simulink model "T7_R2021a"  (R2022a)
settings: Solver=FixedStepAuto  StartTime=0.0  StopTime=10  FixedStep=Ts  RelTol=1e-10  AbsTol=1e-10
model workspace (MATLAB code in the model file):
  | %% Electrical parameters of PMSM motor
  | 
  | P_N = 530; % [W]
  | I_N = 1.5; % [A] (rms)
  | U_N = 220; % [V] (rms, line to line)
  | n_N = 4000; % [rpm]
  | PF_N = 0.9925;
  | n_p=2;
  | V_max = 400; %[V] (rms, line to line)
  | t_r_ref = 1e-3;
  | J = 0.384e-4*5; %kg.m^2
  | 
  | 
  | % Calculations:
  | 
  | % Question 1:
  | w_N = n_N*2*pi/60;
  | psi_R = 20*P_N/(sqrt(2)*pi*n_p*I_N*n_N);
  | L_s = 10*sqrt(3)*U_N*sin(acos(PF_N))/(n_p*n_N*pi*I_N);
  | R_s = sqrt(3)*U_N*PF_N/(3*I_N)-P_N/(3*I_N^2);
  | %% Current Controller
  | Ts = 1e-4;
  | T_L = 0;
  | t_r = 1e-3;
  | w_BW = log(9)/t_r;
  | %E_hat = 1i*w*Psi_R;
  | L_s_hat = 0.010;
  | R_s_hat = 4;
  | R_a = w_BW*L_s_hat - R_s_hat;
  | ki = w_BW*(R_s_hat+R_a);
  | kp = w_BW*L_s_hat;
undefined symbols (not defined in the file or in its folder): b, b_hat, I_max, J_hat, L_M, L_M_hat, L_sigma, L_sigma_hat, magnitude, omega_1_N, psi_R_hat, psi_ref, R_hat, R_R, R_R_hat, V_base, V_LL, w_BWs
libraries: simulink x2
settings Model: Creator=martin  LastModifiedBy=Katrine
settings ModelReferenceCC: EnableRefExpFcnMdlSchedulingChecks=off
settings RTWCC: Description=Generic Real-Time Target

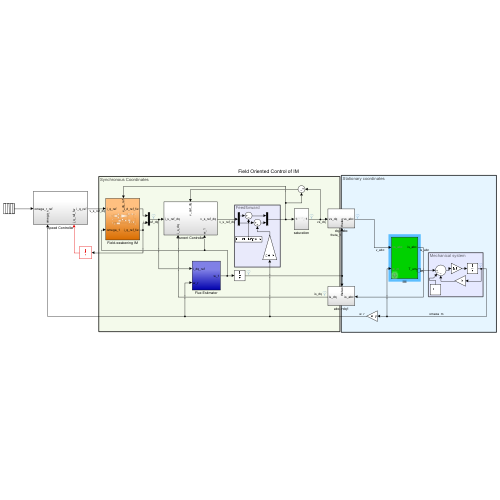
[thumbnail: Simulink's stored preview of the top-level diagram]
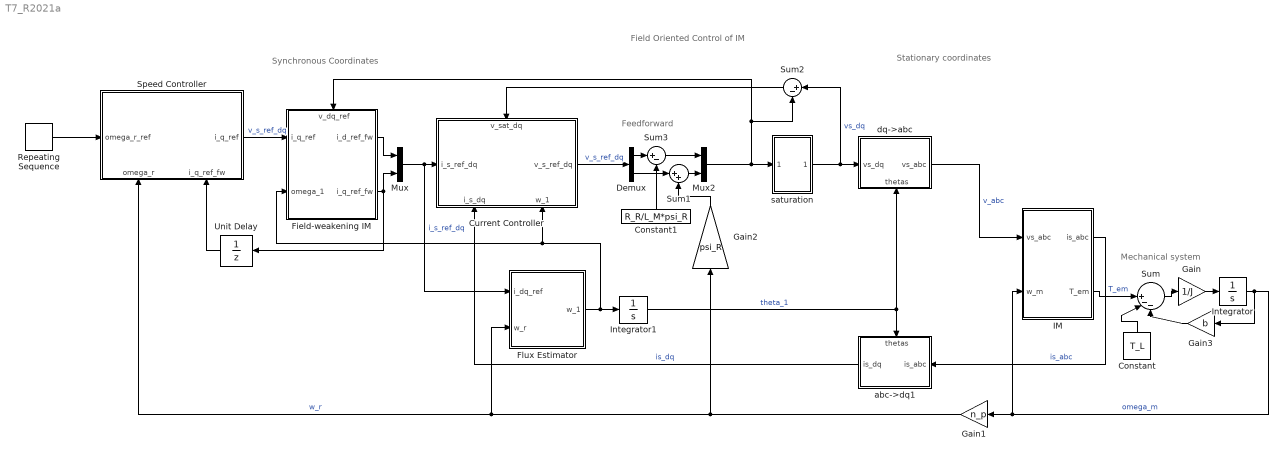
== system T7_R2021a ==
  note: Synchronous Coordinates
  note: Stationary coordinates
  note: Field Oriented Control of IM
  note: Mechanical system
  note: Feedforward
  Constant : Constant  Value=T_L
  Constant1 : Constant  Value=R_R/L_M*psi_R
  Current Controller : Subsystem
      settings: PortSchema="{\"entries\":[{\"content\":{\"sides\":[{\"content\":{\"connectorIds\":[\"In1\"]},\"type\":\"ConnectorPlacement.EquallySpacedRectSide\",\"uuid\":\"97c548b6-6990-4323-a853-1e64e742285c\"},{\"content\":{\"connectorIds\":[\"Out1\"],\"side\":\"RIGHT\"},\"type\":\"ConnectorPlacement.EquallySpacedRectSide\",\"uuid\":\"cacb7644-0a67-4de4-9bb2-887734fe331a\"},{\"content\":{\"connectorIds\":[\"In2\"],\"side\":\"TOP\"},\"type\":\"ConnectorPlacement.EquallySpacedRectSide\",\"uuid\":\"a20c1423-7334-426c-a525-8bdb26886bc3\"},{\"content\":{\"connectorIds\":[\"In3\",\"In4\"],\"side\":\"BOTTOM\"},\"type\":\"ConnectorPlacement.EquallySpacedRectSide\",\"uuid\":\"b9821709-22a3-4c1b-ad46-11760bdb190f\"}]},\"type\":\"ConnectorPlacement.EquallySpacedConnector\",\"uuid\":\"74caaff1-86aa-4f34-8e3a-31d84a5552f1\"}],\"packageUris\":[\"http://schema.mathworks.com/mf0/Connector/R2020b\"],\"version\":\"1.0\"}"
  Demux : Demux  Outputs=2
  Field-weakening IM : Subsystem
      settings: PortSchema="{\"entries\":[{\"content\":{\"sides\":[{\"content\":{\"connectorIds\":[\"In1\",\"In2\"]},\"type\":\"ConnectorPlacement.EquallySpacedRectSide\",\"uuid\":\"aee381d7-3a71-45d0-966d-7af6601206c5\"},{\"content\":{\"connectorIds\":[\"Out1\",\"Out2\"],\"side\":\"RIGHT\"},\"type\":\"ConnectorPlacement.EquallySpacedRectSide\",\"uuid\":\"b4f04b7a-b16d-4ae2-8d18-1ccf45d54418\"},{\"content\":{\"connectorIds\":[\"In3\"],\"side\":\"TOP\"},\"type\":\"ConnectorPlacement.EquallySpacedRectSide\",\"uuid\":\"7d29b16c-0908-4291-9b7c-a89871d4912d\"}]},\"type\":\"ConnectorPlacement.EquallySpacedConnector\",\"uuid\":\"28c927f9-c9f1-4063-8a99-a2da52e20e9b\"}],\"packageUris\":[\"http://schema.mathworks.com/mf0/Connector/R2020b\"],\"version\":\"1.0\"}"
  Flux Estimator : Subsystem
  Gain : Gain  Gain=1/J
  Gain1 : Gain  Gain=n_p
  Gain2 : Gain  Gain=psi_R
  Gain3 : Gain  Gain=b
  IM : Subsystem  mask{R_s=0.5, L_sig=6e-3, R_R=0.312, n_p=1, L_M=0.1}
      mask prompts: R_s "Stator resistance Rs (ohm)"; L_sig "Total leakage inductance L_sig (H)"; R_R "Rotor resistance R_R ( Ohm)"; n_p "Number of pole pairs n_p"; L_M "Magnetising inductance L_M (H)"
      mask help: dynamic model of IM
  Integrator : Integrator  InitialCondition=1337/n_p
  Integrator1 : Integrator
  Mux : Mux  Inputs=2
  Mux2 : Mux  Inputs=2
  Repeating Sequence : simulink/Sources/Repeating Sequence  rep_seq_t=[0 Ts*1e3 5 5+Ts*1e3 10]*1e-3  rep_seq_y=[4.3 4.3 4.3 1 1]
  Speed Controller : Subsystem
      settings: PortSchema="{\"entries\":[{\"content\":{\"sides\":[{\"content\":{\"connectorIds\":[\"In1\"]},\"type\":\"ConnectorPlacement.EquallySpacedRectSide\",\"uuid\":\"97c548b6-6990-4323-a853-1e64e742285c\"},{\"content\":{\"connectorIds\":[\"Out1\"],\"side\":\"RIGHT\"},\"type\":\"ConnectorPlacement.EquallySpacedRectSide\",\"uuid\":\"cacb7644-0a67-4de4-9bb2-887734fe331a\"},{\"content\":{\"connectorIds\":[],\"side\":\"TOP\"},\"type\":\"ConnectorPlacement.EquallySpacedRectSide\",\"uuid\":\"a20c1423-7334-426c-a525-8bdb26886bc3\"},{\"content\":{\"connectorIds\":[\"In2\",\"In3\"],\"side\":\"BOTTOM\"},\"type\":\"ConnectorPlacement.EquallySpacedRectSide\",\"uuid\":\"b9821709-22a3-4c1b-ad46-11760bdb190f\"}]},\"type\":\"ConnectorPlacement.EquallySpacedConnector\",\"uuid\":\"74caaff1-86aa-4f34-8e3a-31d84a5552f1\"}],\"packageUris\":[\"http://schema.mathworks.com/mf0/Connector/R2020b\"],\"version\":\"1.0\"}"
  Sum : Sum  Inputs=||+--
  Sum1 : Sum  Inputs=|++
  Sum2 : Sum  Inputs=|+-
  Sum3 : Sum  Inputs=|+-
  Unit Delay : UnitDelay  InitialCondition=I_max  SampleTime=-1  HasFrameUpgradeWarning=on
  abc->dq1 : Subsystem
      settings: PortSchema="{\"entries\":[{\"content\":{\"sides\":[{\"content\":{\"connectorIds\":[\"In1\"]},\"type\":\"ConnectorPlacement.EquallySpacedRectSide\",\"uuid\":\"c3863cce-4a98-427c-9e63-89298f679a84\"},{\"content\":{\"connectorIds\":[\"Out1\"],\"side\":\"RIGHT\"},\"type\":\"ConnectorPlacement.EquallySpacedRectSide\",\"uuid\":\"ae3c4991-ab62-4114-9bee-e9a7348a29ce\"},{\"content\":{\"connectorIds\":[\"In2\"],\"side\":\"TOP\"},\"type\":\"ConnectorPlacement.EquallySpacedRectSide\",\"uuid\":\"fea582b6-68e0-450b-8231-0f2cf258215e\"},{\"content\":{\"connectorIds\":[],\"side\":\"BOTTOM\"},\"type\":\"ConnectorPlacement.EquallySpacedRectSide\",\"uuid\":\"4cb5cb50-d1c5-41cc-b580-d3f7a61a133b\"}]},\"type\":\"ConnectorPlacement.EquallySpacedConnector\",\"uuid\":\"936995e1-3667-4d5a-83ac-5ed23eb7cec5\"}],\"packageUris\":[\"http://schema.mathworks.com/mf0/Connector/R2020b\"],\"version\":\"1.0\"}"
  dq->abc : Subsystem
      settings: PortSchema="{\"entries\":[{\"content\":{\"sides\":[{\"content\":{\"connectorIds\":[\"In1\"]},\"type\":\"ConnectorPlacement.EquallySpacedRectSide\",\"uuid\":\"c3863cce-4a98-427c-9e63-89298f679a84\"},{\"content\":{\"connectorIds\":[\"Out1\"],\"side\":\"RIGHT\"},\"type\":\"ConnectorPlacement.EquallySpacedRectSide\",\"uuid\":\"ae3c4991-ab62-4114-9bee-e9a7348a29ce\"},{\"content\":{\"connectorIds\":[],\"side\":\"TOP\"},\"type\":\"ConnectorPlacement.EquallySpacedRectSide\",\"uuid\":\"fea582b6-68e0-450b-8231-0f2cf258215e\"},{\"content\":{\"connectorIds\":[\"In2\"],\"side\":\"BOTTOM\"},\"type\":\"ConnectorPlacement.EquallySpacedRectSide\",\"uuid\":\"09df17c4-38be-4fcd-b44b-abaf9d5b2651\"}]},\"type\":\"ConnectorPlacement.EquallySpacedConnector\",\"uuid\":\"936995e1-3667-4d5a-83ac-5ed23eb7cec5\"}],\"packageUris\":[\"http://schema.mathworks.com/mf0/Connector/R2020b\"],\"version\":\"1.0\"}"
  saturation : Subsystem
  wires:
  dq->abc/1(vs_abc) -> IM/1(vs_abc)  "v_abc"
  Sum/1 -> Gain/1
  Gain/1 -> Integrator/1
  Integrator/1 -> Gain3/1, IM/2(w_m), Gain1/1  "omega_m"
  IM/2(T_em) -> Sum/1  "T_em"
  Constant/1 -> Sum/2
  IM/1(is_abc) -> abc->dq1/1(is_abc)  "is_abc"
  Integrator1/1 -> dq->abc/2(thetas), abc->dq1/2(thetas)  "theta_1"
  abc->dq1/1(is_dq) -> Current Controller/3(i_s_dq)  "is_dq"
  Mux/1 -> Flux Estimator/1(i_dq_ref), Current Controller/1(i_s_ref_dq)  "i_s_ref_dq"
  Current Controller/1(v_s_ref_dq) -> Demux/1  "v_s_ref_dq"
  Demux/2 -> Sum1/1
  Sum1/1 -> Mux2/2
  saturation/1(Out1) -> Sum2/1, dq->abc/1(vs_dq)  "vs_dq"
  Gain2/1 -> Sum1/2
  Sum2/1 -> Current Controller/2(v_sat_dq)
  Flux Estimator/1(w_1) -> Field-weakening IM/2(omega_1), Current Controller/4(w_1), Integrator1/1
  Gain1/1 -> Speed Controller/2(omega_r), Flux Estimator/2(w_r), Gain2/1  "w_r"
  Demux/1 -> Sum3/1
  Sum3/1 -> Mux2/1
  Constant1/1 -> Sum3/2
  Field-weakening IM/1(i_d_ref_fw) -> Mux/1
  Field-weakening IM/2(i_q_ref_fw) -> Unit Delay/1, Mux/2
  Mux2/1 -> Field-weakening IM/3(v_dq_ref), Sum2/2, saturation/1(In1)
  Gain3/1 -> Sum/3
  Speed Controller/1(i_q_ref) -> Field-weakening IM/1(i_q_ref)  "v_s_ref_dq"
  Repeating Sequence/1 -> Speed Controller/1(omega_r_ref)
  Unit Delay/1 -> Speed Controller/3(i_q_ref_fw)

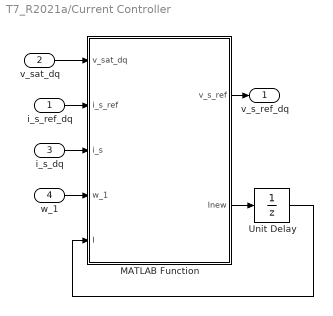
== system T7_R2021a/Current Controller ==
  i_s_ref_dq : Inport
  v_sat_dq : Inport  Port=2
  i_s_dq : Inport  Port=3
  w_1 : Inport  Port=4
  MATLAB Function : MATLAB Function  TreatAsAtomicUnit=on
  Unit Delay : UnitDelay  SampleTime=-1  HasFrameUpgradeWarning=on
  v_s_ref_dq : Outport  PortDimensions=2
  wires:
  MATLAB Function/2(Inew) -> Unit Delay/1
  i_s_ref_dq/1 -> MATLAB Function/2(i_s_ref)
  w_1/1 -> MATLAB Function/4(w_1)
  i_s_dq/1 -> MATLAB Function/3(i_s)
  Unit Delay/1 -> MATLAB Function/5(I)
  MATLAB Function/1(v_s_ref) -> v_s_ref_dq/1
  v_sat_dq/1 -> MATLAB Function/1(v_sat_dq)

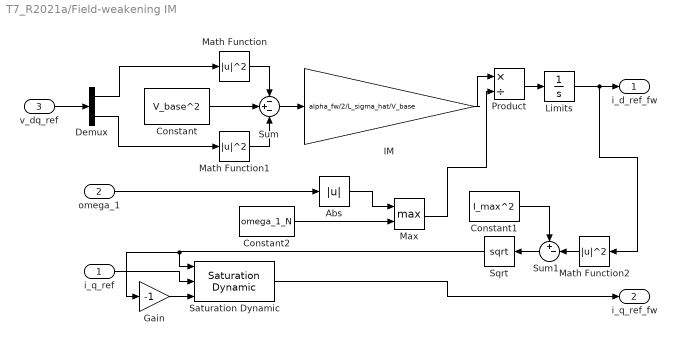
== system T7_R2021a/Field-weakening IM ==
  i_q_ref : Inport
  omega_1 : Inport  Port=2
  v_dq_ref : Inport  Port=3
  Abs : Abs  SaturateOnIntegerOverflow=off
  Constant : Constant  Value=V_base^2
  Constant1 : Constant  Value=I_max^2
  Constant2 : Constant  Value=omega_1_N
  Demux : Demux  Outputs=2
  Gain : Gain  Gain=-1
  IM : Gain  Gain=alpha_fw/2/L_sigma_hat/V_base
  Limits : Integrator  LimitOutput=on  UpperSaturationLimit=psi_ref/L_M_hat  LowerSaturationLimit=0.1*psi_ref/L_M_hat
  Math Function : Math  Operator=magnitude^2
  Math Function1 : Math  Operator=magnitude^2
  Math Function2 : Math  Operator=magnitude^2
  Max : MinMax  Function=max  Inputs=2
  Product : Product  Inputs=*/
  Saturation Dynamic : simulink/Discontinuities/Saturation Dynamic  OutMin=[]  OutMax=[]  OutDataTypeStr=Inherit: Same as second input  OutDataType=fixdt(1, 16)  OutScaling=2^-10  DoSatur=off
  Sqrt : Sqrt
  Sum : Sum  Inputs=-+-
  Sum1 : Sum  Inputs=+-|
  i_d_ref_fw : Outport
  i_q_ref_fw : Outport  Port=2
  wires:
  i_q_ref/1 -> Saturation Dynamic/2
  Constant/1 -> Sum/2
  Math Function/1 -> Sum/1
  Math Function1/1 -> Sum/3
  Sum/1 -> IM/1
  IM/1 -> Product/1
  omega_1/1 -> Abs/1
  Abs/1 -> Max/1
  Max/1 -> Product/2
  Product/1 -> Limits/1
  Limits/1 -> i_d_ref_fw/1, Math Function2/1
  Math Function2/1 -> Sum1/2
  Constant1/1 -> Sum1/1
  Sum1/1 -> Sqrt/1
  Sqrt/1 -> Gain/1, Saturation Dynamic/1
  Gain/1 -> Saturation Dynamic/3
  Saturation Dynamic/1 -> i_q_ref_fw/1
  Constant2/1 -> Max/2
  v_dq_ref/1 -> Demux/1
  Demux/1 -> Math Function/1
  Demux/2 -> Math Function1/1

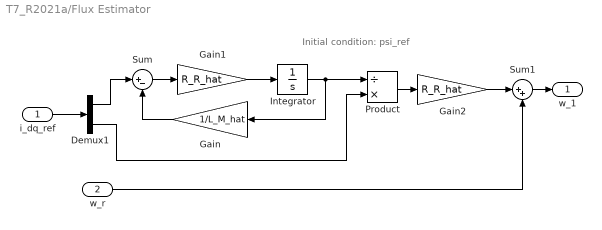
== system T7_R2021a/Flux Estimator ==
  note: Initial condition: psi_ref
  i_dq_ref : Inport
  w_r : Inport  Port=2
  Demux1 : Demux  Outputs=2
  Gain : Gain  Gain=1/L_M_hat
  Gain1 : Gain  Gain=R_R_hat
  Gain2 : Gain  Gain=R_R_hat
  Integrator : Integrator  InitialCondition=psi_ref
  Product : Product  Inputs=/*
  Sum : Sum  Inputs=|+-
  Sum1 : Sum  Inputs=|++
  w_1 : Outport
  wires:
  w_r/1 -> Sum1/2
  Sum1/1 -> w_1/1
  Gain2/1 -> Sum1/1
  Product/1 -> Gain2/1
  Demux1/2 -> Product/2
  Gain1/1 -> Integrator/1
  Sum/1 -> Gain1/1
  Gain/1 -> Sum/2
  Integrator/1 -> Gain/1, Product/1
  i_dq_ref/1 -> Demux1/1
  Demux1/1 -> Sum/1

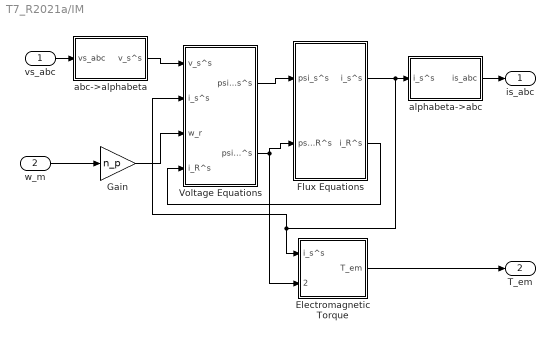
== system T7_R2021a/IM ==
  vs_abc : Inport
  w_m : Inport  Port=2
  Electromagnetic Torque : Subsystem
  Flux Equations : Subsystem
  Gain : Gain  Gain=n_p  SaturateOnIntegerOverflow=on  OutDataTypeStr=Inherit: Same as input  ParamDataTypeStr=Inherit: Same as input
  Voltage Equations : Subsystem
  abc->alphabeta : Subsystem
  alphabeta->abc : Subsystem
  is_abc : Outport
  T_em : Outport  Port=2
  wires:
  Gain/1 -> Voltage Equations/3(w_r)
  alphabeta->abc/1(is_abc) -> is_abc/1
  abc->alphabeta/1(v_s^s) -> Voltage Equations/1(v_s^s)
  Voltage Equations/1(psi_s^s) -> Flux Equations/1(psi_s^s)
  Voltage Equations/2(psi_R^s) -> Flux Equations/2(psi_R^s), Electromagnetic Torque/2(psi_R^s)
  vs_abc/1 -> abc->alphabeta/1(vs_abc)
  Flux Equations/1(i_s^s) -> Electromagnetic Torque/1(i_s^s), Voltage Equations/2(i_s^s), alphabeta->abc/1(i_s^s)
  Electromagnetic Torque/1(T_em) -> T_em/1
  w_m/1 -> Gain/1
  Flux Equations/2(i_R^s) -> Voltage Equations/4(i_R^s)

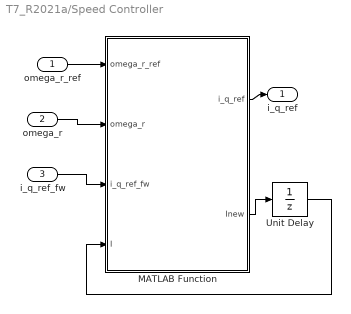
== system T7_R2021a/Speed Controller ==
  omega_r_ref : Inport
  omega_r : Inport  Port=2
  i_q_ref_fw : Inport  Port=3
  MATLAB Function : MATLAB Function  TreatAsAtomicUnit=on
  Unit Delay : UnitDelay  SampleTime=-1  HasFrameUpgradeWarning=on
  i_q_ref : Outport  PortDimensions=2
  wires:
  MATLAB Function/2(Inew) -> Unit Delay/1
  omega_r/1 -> MATLAB Function/2(omega_r)
  Unit Delay/1 -> MATLAB Function/4(I)
  MATLAB Function/1(i_q_ref) -> i_q_ref/1
  omega_r_ref/1 -> MATLAB Function/1(omega_r_ref)
  i_q_ref_fw/1 -> MATLAB Function/3(i_q_ref_fw)

== system T7_R2021a/abc->dq1 ==
  is_abc : Inport
  thetas : Inport  Port=2
  MATLAB Function : MATLAB Function  TreatAsAtomicUnit=on
  is_dq : Outport
  wires:
  MATLAB Function/1(is) -> is_dq/1
  thetas/1 -> MATLAB Function/2(thetas)
  is_abc/1 -> MATLAB Function/1(is_abc)

== system T7_R2021a/dq->abc ==
  vs_dq : Inport
  thetas : Inport  Port=2
  MATLAB Function : MATLAB Function  TreatAsAtomicUnit=on
  vs_abc : Outport
  wires:
  MATLAB Function/1(vs_abc) -> vs_abc/1
  thetas/1 -> MATLAB Function/2(thetas)
  vs_dq/1 -> MATLAB Function/1(vs_dq)

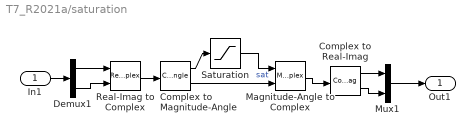
== system T7_R2021a/saturation ==
  In1 : Inport
  Complex to Magnitude-Angle : ComplexToMagnitudeAngle
  Complex to Real-Imag : ComplexToRealImag
  Demux1 : Demux  Outputs=2
  Magnitude-Angle to Complex : MagnitudeAngleToComplex
  Mux1 : Mux  Inputs=2
  Real-Imag to Complex : RealImagToComplex
  Saturation : Saturate  UpperLimit=V_LL*sqrt(2)/sqrt(3)  LowerLimit=0
  Out1 : Outport
  wires:
  Mux1/1 -> Out1/1
  Demux1/2 -> Real-Imag to Complex/2
  Complex to Real-Imag/1 -> Mux1/1
  Magnitude-Angle to Complex/1 -> Complex to Real-Imag/1
  Demux1/1 -> Real-Imag to Complex/1
  Real-Imag to Complex/1 -> Complex to Magnitude-Angle/1
  Complex to Real-Imag/2 -> Mux1/2
  In1/1 -> Demux1/1
  Complex to Magnitude-Angle/1 -> Saturation/1
  Saturation/1 -> Magnitude-Angle to Complex/1  "sat"
  Complex to Magnitude-Angle/2 -> Magnitude-Angle to Complex/2

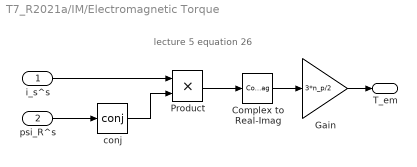
== system T7_R2021a/IM/Electromagnetic Torque ==
  note: lecture 5 equation 26
  i_s^s : Inport
  psi_R^s : Inport  Port=2
  Complex to Real-Imag : ComplexToRealImag  Output=Imag
  Gain : Gain  Gain=3*n_p/2
  Product : Product
  conj : Math  Operator=conj
  T_em : Outport
  wires:
  psi_R^s/1 -> conj/1
  i_s^s/1 -> Product/1
  conj/1 -> Product/2
  Product/1 -> Complex to Real-Imag/1
  Complex to Real-Imag/1 -> Gain/1
  Gain/1 -> T_em/1

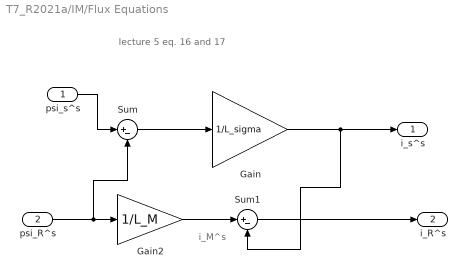
== system T7_R2021a/IM/Flux Equations ==
  note: i_M^s
  note: lecture 5 eq. 16 and 17
  psi_s^s : Inport
  psi_R^s : Inport  Port=2
  Gain : Gain  Gain=1/L_sigma
  Gain2 : Gain  Gain=1/L_M
  Sum : Sum  Inputs=|+-
  Sum1 : Sum  Inputs=|+-
  i_s^s : Outport
  i_R^s : Outport  Port=2
  wires:
  psi_s^s/1 -> Sum/1
  Sum/1 -> Gain/1
  psi_R^s/1 -> Sum/2, Gain2/1
  Gain2/1 -> Sum1/1
  Gain/1 -> i_s^s/1, Sum1/2
  Sum1/1 -> i_R^s/1

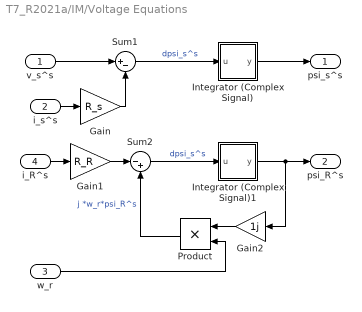
== system T7_R2021a/IM/Voltage Equations ==
  v_s^s : Inport
  i_s^s : Inport  Port=2
  w_r : Inport  Port=3
  i_R^s : Inport  Port=4
  Gain : Gain  Gain=R_s
  Gain1 : Gain  Gain=R_R
  Gain2 : Gain  Gain=1j
  Integrator (Complex Signal) : Subsystem
      mask Display: disp('1/s');
  Integrator (Complex Signal)1 : Subsystem
      mask Display: disp('1/s');
  Product : Product  RndMeth=Zero
  Sum1 : Sum  Inputs=|+-
  Sum2 : Sum  Inputs=|-+
  psi_s^s : Outport
  psi_R^s : Outport  Port=2
  wires:
  w_r/1 -> Product/2
  Gain2/1 -> Product/1
  Integrator (Complex Signal)1/1(y) -> Gain2/1, psi_R^s/1
  Integrator (Complex Signal)/1(y) -> psi_s^s/1
  Gain/1 -> Sum1/2
  Sum1/1 -> Integrator (Complex Signal)/1(u)  "dpsi_s^s"
  i_s^s/1 -> Gain/1
  v_s^s/1 -> Sum1/1
  Product/1 -> Sum2/2  "j *w_r*psi_R^s"
  i_R^s/1 -> Gain1/1
  Gain1/1 -> Sum2/1
  Sum2/1 -> Integrator (Complex Signal)1/1(u)  "dpsi_s^s"

== system T7_R2021a/IM/abc->alphabeta ==
  vs_abc : Inport
  Fcn : Fcn  Expr=2/3*(u(1)-0.5*u(2)-0.5*u(3))
  Fcn1 : Fcn  Expr=sqrt(3)/3*(u(2)-u(3))
  Real-Imag to Complex : RealImagToComplex
  v_s^s : Outport
  wires:
  Real-Imag to Complex/1 -> v_s^s/1
  Fcn1/1 -> Real-Imag to Complex/2  "beta"
  Fcn/1 -> Real-Imag to Complex/1  "alpha"
  vs_abc/1 -> Fcn/1, Fcn1/1

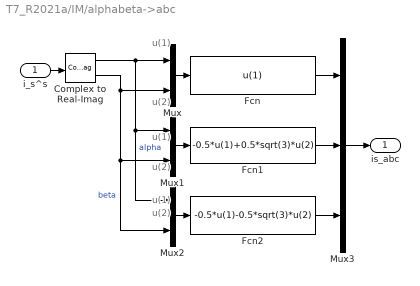
== system T7_R2021a/IM/alphabeta->abc ==
  note: u(2)
  note: u(1)
  note: u(2)
  note: u(1)
  note: u(2)
  note: u(1)
  i_s^s : Inport
  Complex to Real-Imag : ComplexToRealImag
  Fcn : Fcn  Expr=u(1)
  Fcn1 : Fcn  Expr=-0.5*u(1)+0.5*sqrt(3)*u(2)
  Fcn2 : Fcn  Expr=-0.5*u(1)-0.5*sqrt(3)*u(2)
  Mux : Mux  Inputs=2
  Mux1 : Mux  Inputs=2
  Mux2 : Mux  Inputs=2
  Mux3 : Mux  Inputs=3
  is_abc : Outport
  wires:
  Mux3/1 -> is_abc/1
  Fcn2/1 -> Mux3/3
  Fcn1/1 -> Mux3/2
  Fcn/1 -> Mux3/1
  i_s^s/1 -> Complex to Real-Imag/1
  Mux2/1 -> Fcn2/1
  Mux1/1 -> Fcn1/1
  Complex to Real-Imag/2 -> Mux2/2, Mux1/2, Mux/2  "beta"
  Complex to Real-Imag/1 -> Mux2/1, Mux1/1, Mux/1  "alpha"
  Mux/1 -> Fcn/1

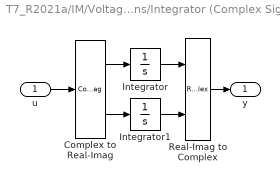
== system T7_R2021a/IM/Voltage Equations/Integrator (Complex Signal) ==
  u : Inport
  Complex to Real-Imag : ComplexToRealImag
  Integrator : Integrator  InitialCondition=psi_ref
  Integrator1 : Integrator
  Real-Imag to Complex : RealImagToComplex
  y : Outport
  wires:
  u/1 -> Complex to Real-Imag/1
  Real-Imag to Complex/1 -> y/1
  Integrator1/1 -> Real-Imag to Complex/2
  Integrator/1 -> Real-Imag to Complex/1
  Complex to Real-Imag/2 -> Integrator1/1
  Complex to Real-Imag/1 -> Integrator/1

== system T7_R2021a/IM/Voltage Equations/Integrator (Complex Signal)1 ==
  u : Inport
  Complex to Real-Imag : ComplexToRealImag
  Integrator : Integrator  InitialCondition=psi_ref
  Integrator1 : Integrator
  Real-Imag to Complex : RealImagToComplex
  y : Outport
  wires:
  u/1 -> Complex to Real-Imag/1
  Real-Imag to Complex/1 -> y/1
  Integrator1/1 -> Real-Imag to Complex/2
  Integrator/1 -> Real-Imag to Complex/1
  Complex to Real-Imag/2 -> Integrator1/1
  Complex to Real-Imag/1 -> Integrator/1

== matlab function T7_R2021a/dq->abc/MATLAB Function ==
  data: vs_dq input size=2; thetas input size=1; vs_abc output size=3
function vs_abc = dq_abc(vs_dq, thetas)
%#codegen

% voltage in synchronous coordinates:
 vd = vs_dq(1); vq = vs_dq(2); 
vs_dq = [vd;vq];

% coordinate transformation and Space-vector transformation 
T_alphabeta = [cos(thetas), -sin(thetas); sin(thetas), cos(thetas)];
T_23 = [1, 0; -1/2, sqrt(3)/2; -1/2, -sqrt(3)/2];
vs_abc = T_23*T_alphabeta*vs_dq;   % Complete this

== matlab function T7_R2021a/Speed Controller/MATLAB Function ==
  data: omega_r_ref input size=2; omega_r input size=2; i_q_ref_fw input; I input size=1; w_BWs parameter size=1; i_q_ref output size=2; Inew output; psi_R_hat parameter size=1; J_hat parameter size=1; Ts parameter; b_hat parameter; I_max parameter; n_p parameter
function [i_q_ref, Inew] = sc(omega_r_ref, omega_r, i_q_ref_fw,I, w_BWs, psi_R_hat, J_hat, Ts, b_hat, I_max, n_p)
%#codegen

%% Current controller 
% Gains
kps = 2*J_hat*w_BWs/(3*n_p^2*psi_R_hat); % notes psi_R_hat is psi_ref
kis = w_BWs^2*2*J_hat/(3*n_p^2*psi_R_hat); % notes
ba = 2*J_hat/(3*n_p^2*psi_R_hat)*(w_BWs-b_hat/J_hat); % notes
e = omega_r_ref - omega_r;
i_q_ref_nom = kps*e+kis*I-ba*omega_r; % complete: PI + active damping ba, real
i_q_ref = i_q_ref_fw;

%% Update the integral state of the speed controller 
Inew = I + Ts*(e + (i_q_ref - i_q_ref_nom)/kps);

== matlab function T7_R2021a/abc->dq1/MATLAB Function ==
  data: is_abc input size=3; thetas input size=1; is output size=2
function is = abc_dq(is_abc, thetas)
%#codegen

% Phase currents
ia = is_abc(1); ib = is_abc(2); ic = is_abc(3); 
is_abc = [ia;ib;ic];
% Space-vector transformation and coordinate transformation
T_dq = [cos(thetas), sin(thetas); -sin(thetas), cos(thetas)];
T_32 = [2/3, -1/3, -1/3; 0, 1/sqrt(3), -1/sqrt(3)];
is = T_dq*T_32*is_abc;   % Complete this

== matlab function T7_R2021a/Current Controller/MATLAB Function ==
  data: v_sat_dq input size=2; i_s_ref input size=2; i_s input size=2; w_1 input size=1; I input size=1; w_BW parameter size=1; v_s_ref output size=2; Inew output; R_hat parameter size=1; L_sigma_hat parameter size=1; Ts parameter
function [v_s_ref, Inew] = cc(v_sat_dq,i_s_ref, i_s, w_1, I, w_BW, R_hat, L_sigma_hat, Ts)
%#codegen

%% Current controller 
% Gains
kp = w_BW*L_sigma_hat; % L7 p15
ki = w_BW^2*L_sigma_hat; % L7 p15
Ra = w_BW*L_sigma_hat - R_hat; % L7 p14

% Voltage reference in synchronous coordinates
i_s = i_s(1)+ 1i*i_s(2);
i_s_ref = i_s_ref(1)+ 1i*i_s_ref(2);
e = i_s_ref - i_s;
% L7 p13 and p15 (c for complex number)
v_s_ref_c = kp*e+ki*I + 1i*w_1*L_sigma_hat*i_s_ref-Ra*i_s_ref; % complete: PI + active resistance Ra + decoupler.
v_s_ref = [real(v_s_ref_c);imag(v_s_ref_c)];

%% Update the integral state of the current controller 
v_sat_dq_c = v_sat_dq(1)+ 1i*v_sat_dq(2);
Inew = I + Ts*(e + (v_sat_dq_c)/kp);
